simulink model "PX4_Run_Mode_R2017b"  (R2017b)
settings: Solver=FixedStepDiscrete  StartTime=0.0  StopTime=10.0  RelTol=1e-3  EnableMultiTasking=on
InitFcn:
  | run('InitFcn_R2017b_no_csc.m');
values from neighbouring files (symbols this model uses):
  A = Pixhawk_CSC.Parameter( {single([diag([1 1 1]) Ts*diag([1 1 1]); diag([0 0 0]) diag([1 1 1])]),'A'} )    [InitFcn.m]    (also in InitFcn_R2016b.m; InitFcn_R2017b_no_csc.m = single([diag([1 1 1]) Ts*diag([1 1 1]); diag([0 0 0]) diag([)
  app = Pixhawk_CSC.Parameter({single( [0.05; 0.05; 0.05]),'app'} )    [InitFcn.m]    (also in InitFcn_R2016b.m; InitFcn_R2017b_no_csc.m = single( [0.05; 0.05; 0.05]))
  B = Pixhawk_CSC.Parameter( {single([Ts^2/2*diag([1 1 1]); Ts*diag([1 1 1])]),'B'} )    [InitFcn.m]    (also in InitFcn_R2016b.m; InitFcn_R2017b_no_csc.m = single([Ts^2/2*diag([1 1 1]); Ts*diag([1 1 1])]))
  Beta = Pixhawk_CSC.Parameter({single( 0.02),'Beta'} )    [InitFcn.m]    (also in InitFcn_R2016b.m; InitFcn_R2017b_no_csc.m = single( 0.02))
  C = Pixhawk_CSC.Parameter( {single([diag([1 1 1]) 0*diag([1 1 1]); zeros(1,2) 1 zeros(1,3)]),'C'} )    [InitFcn.m]    (also in InitFcn_R2016b.m; InitFcn_R2017b_no_csc.m = single([diag([1 1 1]) 0*diag([1 1 1]); zeros(1,2) 1 zeros(1,)
  C1 = Pixhawk_CSC.Parameter({single( 1.08680),'C1'} )    [InitFcn.m]    (also in InitFcn_R2016b.m; InitFcn_R2017b_no_csc.m = single( 1.08680))
  C10 = Pixhawk_CSC.Parameter({single( 0.0000),'C10'} )    [InitFcn.m]    (also in InitFcn_R2016b.m; InitFcn_R2017b_no_csc.m = single( 0.0000))
  C11 = Pixhawk_CSC.Parameter({single(-0.2300),'C11'} )    [InitFcn.m]    (also in InitFcn_R2016b.m; InitFcn_R2017b_no_csc.m = single(-0.2300))
  C12 = Pixhawk_CSC.Parameter({single( 0.0000),'C12'} )    [InitFcn.m]    (also in InitFcn_R2016b.m; InitFcn_R2017b_no_csc.m = single( 0.0000))
  C13 = Pixhawk_CSC.Parameter({single( 0.8000),'C13'} )    [InitFcn.m]    (also in InitFcn_R2016b.m; InitFcn_R2017b_no_csc.m = single( 0.8000))
  C14 = Pixhawk_CSC.Parameter({single( 0.8000),'C14'} )    [InitFcn.m]    (also in InitFcn_R2016b.m; InitFcn_R2017b_no_csc.m = single( 0.8000))
  C15 = Pixhawk_CSC.Parameter({single( 1.73200),'C15'} )    [InitFcn.m]    (also in InitFcn_R2016b.m; InitFcn_R2017b_no_csc.m = single( 1.73200))
  C16 = Pixhawk_CSC.Parameter({single( 0.1000),'C16'} )    [InitFcn.m]    (also in InitFcn_R2016b.m; InitFcn_R2017b_no_csc.m = single( 0.1000))
  C17 = Pixhawk_CSC.Parameter({single( 0.1000),'C17'} )    [InitFcn.m]    (also in InitFcn_R2016b.m; InitFcn_R2017b_no_csc.m = single( 0.1000))
  C18 = Pixhawk_CSC.Parameter({single( 0.0500),'C18'} )    [InitFcn.m]    (also in InitFcn_R2016b.m; InitFcn_R2017b_no_csc.m = single( 0.0500))
  C19 = Pixhawk_CSC.Parameter({single( 0.6000),'C19'} )    [InitFcn.m]    (also in InitFcn_R2016b.m; InitFcn_R2017b_no_csc.m = single( 0.6000))
  C2 = Pixhawk_CSC.Parameter({single( 1.10468),'C2'} )    [InitFcn.m]    (also in InitFcn_R2016b.m; InitFcn_R2017b_no_csc.m = single( 1.10468))
  C20 = Pixhawk_CSC.Parameter({single( 0.6000),'C20'} )    [InitFcn.m]    (also in InitFcn_R2016b.m; InitFcn_R2017b_no_csc.m = single( 0.6000))
  C21 = Pixhawk_CSC.Parameter({single( 1.04558),'C21'} )    [InitFcn.m]    (also in InitFcn_R2016b.m; InitFcn_R2017b_no_csc.m = single( 1.04558))
  C22 = Pixhawk_CSC.Parameter({single( 0.0000),'C22'} )    [InitFcn.m]    (also in InitFcn_R2016b.m; InitFcn_R2017b_no_csc.m = single( 0.0000))
  C23 = Pixhawk_CSC.Parameter({single( 0.0000),'C23'} )    [InitFcn.m]    (also in InitFcn_R2016b.m; InitFcn_R2017b_no_csc.m = single( 0.0000))
  C24 = Pixhawk_CSC.Parameter({single(-11.0000),'C24'} )    [InitFcn.m]    (also in InitFcn_R2016b.m; InitFcn_R2017b_no_csc.m = single(-11.0000))
  C3 = Pixhawk_CSC.Parameter({single( 1.1980),'C3'} )    [InitFcn.m]    (also in InitFcn_R2016b.m; InitFcn_R2017b_no_csc.m = single( 1.1980))
  C4 = Pixhawk_CSC.Parameter({single( 0.0500),'C4'} )    [InitFcn.m]    (also in InitFcn_R2016b.m; InitFcn_R2017b_no_csc.m = single( 0.0500))
  C5 = Pixhawk_CSC.Parameter({single( 0.0500),'C5'} )    [InitFcn.m]    (also in InitFcn_R2016b.m; InitFcn_R2017b_no_csc.m = single( 0.0500))
  C6 = Pixhawk_CSC.Parameter({single( 0.0500),'C6'} )    [InitFcn.m]    (also in InitFcn_R2016b.m; InitFcn_R2017b_no_csc.m = single( 0.0500))
  C7 = Pixhawk_CSC.Parameter({single( 0.35937),'C7'} )    [InitFcn.m]    (also in InitFcn_R2016b.m; InitFcn_R2017b_no_csc.m = single( 0.35937))
  C8 = Pixhawk_CSC.Parameter({single( 0.36528),'C8'} )    [InitFcn.m]    (also in InitFcn_R2016b.m; InitFcn_R2017b_no_csc.m = single( 0.36528))
  C9 = Pixhawk_CSC.Parameter({single( 0.53311),'C9'} )    [InitFcn.m]    (also in InitFcn_R2016b.m; InitFcn_R2017b_no_csc.m = single( 0.53311))
  C_1 = Pixhawk_CSC.Parameter( {single([diag([1 1 1]) 0*diag([1 1 1])]),'C1'} )    [InitFcn.m]    (also in InitFcn_R2016b.m; InitFcn_R2017b_no_csc.m = single([diag([1 1 1]) 0*diag([1 1 1])]))
  CAL_ACC0_XOFFSET = Pixhawk_CSC.Parameter( {single( 0.122052  ),'CAL_ACC0_XOFFSET'} )    [InitFcn.m]    (also in InitFcn_R2016b.m; InitFcn_R2017b_no_csc.m = single( 0.122052  ))
  CAL_ACC0_XXSCALE = Pixhawk_CSC.Parameter( {single(  1.01218    ),'CAL_ACC0_XXSCALE'} )    [InitFcn.m]    (also in InitFcn_R2016b.m; InitFcn_R2017b_no_csc.m = single(  1.01218    ))
  CAL_ACC0_XYSCALE = Pixhawk_CSC.Parameter( {single( -0.00443301 ),'CAL_ACC0_XYSCALE'} )    [InitFcn.m]    (also in InitFcn_R2016b.m; InitFcn_R2017b_no_csc.m = single( -0.00443301 ))
  CAL_ACC0_XZSCALE = Pixhawk_CSC.Parameter( {single( -0.00505793 ),'CAL_ACC0_XZSCALE'} )    [InitFcn.m]    (also in InitFcn_R2016b.m; InitFcn_R2017b_no_csc.m = single( -0.00505793 ))
  CAL_ACC0_YOFFSET = Pixhawk_CSC.Parameter( {single( 0.00281205),'CAL_ACC0_YOFFSET'} )    [InitFcn.m]    (also in InitFcn_R2016b.m; InitFcn_R2017b_no_csc.m = single( 0.00281205))
  CAL_ACC0_YXSCALE = Pixhawk_CSC.Parameter( {single( -0.00443301 ),'CAL_ACC0_YXSCALE'} )    [InitFcn.m]    (also in InitFcn_R2016b.m; InitFcn_R2017b_no_csc.m = single( -0.00443301 ))
  CAL_ACC0_YYSCALE = Pixhawk_CSC.Parameter( {single(  1.00234    ),'CAL_ACC0_YYSCALE'} )    [InitFcn.m]    (also in InitFcn_R2016b.m; InitFcn_R2017b_no_csc.m = single(  1.00234    ))
  CAL_ACC0_YZSCALE = Pixhawk_CSC.Parameter( {single(  0.0160883  ),'CAL_ACC0_YZSCALE'} )    [InitFcn.m]    (also in InitFcn_R2016b.m; InitFcn_R2017b_no_csc.m = single(  0.0160883  ))
  CAL_ACC0_ZOFFSET = Pixhawk_CSC.Parameter( {single(-0.0298121 ),'CAL_ACC0_ZOFFSET'} )    [InitFcn.m]    (also in InitFcn_R2016b.m; InitFcn_R2017b_no_csc.m = single(-0.0298121 ))
  CAL_ACC0_ZXSCALE = Pixhawk_CSC.Parameter( {single( -0.00505793 ),'CAL_ACC0_ZXSCALE'} )    [InitFcn.m]    (also in InitFcn_R2016b.m; InitFcn_R2017b_no_csc.m = single( -0.00505793 ))
  CAL_ACC0_ZYSCALE = Pixhawk_CSC.Parameter( {single(  0.0160883  ),'CAL_ACC0_ZYSCALE'} )    [InitFcn.m]    (also in InitFcn_R2016b.m; InitFcn_R2017b_no_csc.m = single(  0.0160883  ))
  CAL_ACC0_ZZSCALE = Pixhawk_CSC.Parameter( {single(  0.983604   ),'CAL_ACC0_ZZSCALE'} )    [InitFcn.m]    (also in InitFcn_R2016b.m; InitFcn_R2017b_no_csc.m = single(  0.983604   ))
  CAL_BAR_OFFSET = Pixhawk_CSC.Parameter( {single( -20.8468),'CAL_BAR_OFFSET'} )    [InitFcn.m]    (also in InitFcn_R2016b.m; InitFcn_R2017b_no_csc.m = single( -20.8468))
  CAL_BAR_SCALE = Pixhawk_CSC.Parameter( {single(   1.0632),'CAL_BAR_SCALE'} )    [InitFcn.m]    (also in InitFcn_R2016b.m; InitFcn_R2017b_no_csc.m = single(   1.0632))
  CAL_BAT0_XOFFSET = Pixhawk_CSC.Parameter( {single( 0.0000),'CAL_BAT0_XOFFSET'} )    [InitFcn.m]    (also in InitFcn_R2016b.m; InitFcn_R2017b_no_csc.m = single( 0.0000))
  CAL_BAT0_XXSCALE = Pixhawk_CSC.Parameter( {single(  1.0000),'CAL_BAT0_XXSCALE'} )    [InitFcn.m]    (also in InitFcn_R2016b.m; InitFcn_R2017b_no_csc.m = single(  1.0000))
  CAL_BAT0_XYSCALE = Pixhawk_CSC.Parameter( {single(  0.0000),'CAL_BAT0_XYSCALE'} )    [InitFcn.m]    (also in InitFcn_R2016b.m; InitFcn_R2017b_no_csc.m = single(  0.0000))
  CAL_BAT0_XZSCALE = Pixhawk_CSC.Parameter( {single(  0.0000),'CAL_BAT0_XZSCALE'} )    [InitFcn.m]    (also in InitFcn_R2016b.m; InitFcn_R2017b_no_csc.m = single(  0.0000))
  CAL_BAT0_YOFFSET = Pixhawk_CSC.Parameter( {single( 0.0000),'CAL_BAT0_YOFFSET'} )    [InitFcn.m]    (also in InitFcn_R2016b.m; InitFcn_R2017b_no_csc.m = single( 0.0000))
  CAL_BAT0_YXSCALE = Pixhawk_CSC.Parameter( {single(  0.0000),'CAL_BAT0_YXSCALE'} )    [InitFcn.m]    (also in InitFcn_R2016b.m; InitFcn_R2017b_no_csc.m = single(  0.0000))
  CAL_BAT0_YYSCALE = Pixhawk_CSC.Parameter( {single(  1.0000),'CAL_BAT0_YYSCALE'} )    [InitFcn.m]    (also in InitFcn_R2016b.m; InitFcn_R2017b_no_csc.m = single(  1.0000))
  CAL_BAT0_YZSCALE = Pixhawk_CSC.Parameter( {single(  0.0000),'CAL_BAT0_YZSCALE'} )    [InitFcn.m]    (also in InitFcn_R2016b.m; InitFcn_R2017b_no_csc.m = single(  0.0000))
  CAL_BAT0_ZOFFSET = Pixhawk_CSC.Parameter( {single( 0.0000),'CAL_BAT0_ZOFFSET'} )    [InitFcn.m]    (also in InitFcn_R2016b.m; InitFcn_R2017b_no_csc.m = single( 0.0000))
  CAL_BAT0_ZXSCALE = Pixhawk_CSC.Parameter( {single(  0.0000),'CAL_BAT0_ZXSCALE'} )    [InitFcn.m]    (also in InitFcn_R2016b.m; InitFcn_R2017b_no_csc.m = single(  0.0000))
  CAL_BAT0_ZYSCALE = Pixhawk_CSC.Parameter( {single(  0.0000),'CAL_BAT0_ZYSCALE'} )    [InitFcn.m]    (also in InitFcn_R2016b.m; InitFcn_R2017b_no_csc.m = single(  0.0000))
  CAL_BAT0_ZZSCALE = Pixhawk_CSC.Parameter( {single(  1.0000),'CAL_BAT0_ZZSCALE'} )    [InitFcn.m]    (also in InitFcn_R2016b.m; InitFcn_R2017b_no_csc.m = single(  1.0000))
  CAL_GPS0_XOFFSET = Pixhawk_CSC.Parameter( {single( 0.0000),'CAL_GPS0_XOFFSET'} )    [InitFcn.m]    (also in InitFcn_R2016b.m; InitFcn_R2017b_no_csc.m = single( 0.0000))
  CAL_GPS0_XXSCALE = Pixhawk_CSC.Parameter( {single(  0.0100),'CAL_GPS0_XXSCALE'} )    [InitFcn.m]    (also in InitFcn_R2016b.m; InitFcn_R2017b_no_csc.m = single(  0.0100))
  CAL_GPS0_XYSCALE = Pixhawk_CSC.Parameter( {single(  0.0000),'CAL_GPS0_XYSCALE'} )    [InitFcn.m]    (also in InitFcn_R2016b.m; InitFcn_R2017b_no_csc.m = single(  0.0000))
  CAL_GPS0_XZSCALE = Pixhawk_CSC.Parameter( {single(  0.0000),'CAL_GPS0_XZSCALE'} )    [InitFcn.m]    (also in InitFcn_R2016b.m; InitFcn_R2017b_no_csc.m = single(  0.0000))
  CAL_GPS0_YOFFSET = Pixhawk_CSC.Parameter( {single( 0.0000),'CAL_GPS0_YOFFSET'} )    [InitFcn.m]    (also in InitFcn_R2016b.m; InitFcn_R2017b_no_csc.m = single( 0.0000))
  CAL_GPS0_YXSCALE = Pixhawk_CSC.Parameter( {single(  0.0000),'CAL_GPS0_YXSCALE'} )    [InitFcn.m]    (also in InitFcn_R2016b.m; InitFcn_R2017b_no_csc.m = single(  0.0000))
  CAL_GPS0_YYSCALE = Pixhawk_CSC.Parameter( {single(  0.0100),'CAL_GPS0_YYSCALE'} )    [InitFcn.m]    (also in InitFcn_R2016b.m; InitFcn_R2017b_no_csc.m = single(  0.0100))
  CAL_GPS0_YZSCALE = Pixhawk_CSC.Parameter( {single(  0.0000),'CAL_GPS0_YZSCALE'} )    [InitFcn.m]    (also in InitFcn_R2016b.m; InitFcn_R2017b_no_csc.m = single(  0.0000))
  CAL_GPS0_ZOFFSET = Pixhawk_CSC.Parameter( {single( 0.0000),'CAL_GPS0_ZOFFSET'} )    [InitFcn.m]    (also in InitFcn_R2016b.m; InitFcn_R2017b_no_csc.m = single( 0.0000))
  CAL_GPS0_ZXSCALE = Pixhawk_CSC.Parameter( {single(  0.0000),'CAL_GPS0_ZXSCALE'} )    [InitFcn.m]    (also in InitFcn_R2016b.m; InitFcn_R2017b_no_csc.m = single(  0.0000))
  CAL_GPS0_ZYSCALE = Pixhawk_CSC.Parameter( {single(  0.0000),'CAL_GPS0_ZYSCALE'} )    [InitFcn.m]    (also in InitFcn_R2016b.m; InitFcn_R2017b_no_csc.m = single(  0.0000))
  CAL_GPS0_ZZSCALE = Pixhawk_CSC.Parameter( {single( -0.0010),'CAL_GPS0_ZZSCALE'} )    [InitFcn.m]    (also in InitFcn_R2016b.m; InitFcn_R2017b_no_csc.m = single( -0.0010))
  CAL_GYRO0_XXSCALE = Pixhawk_CSC.Parameter( {single(0.992736),'CAL_GYRO0_XXSCALE'} )    [InitFcn.m]    (also in InitFcn_R2016b.m; InitFcn_R2017b_no_csc.m = single(0.992736))
  CAL_GYRO0_XYSCALE = Pixhawk_CSC.Parameter( {single(0.0000),'CAL_GYRO0_XYSCALE'} )    [InitFcn.m]    (also in InitFcn_R2016b.m; InitFcn_R2017b_no_csc.m = single(0.0000))
  CAL_GYRO0_XZSCALE = Pixhawk_CSC.Parameter( {single(0.0000),'CAL_GYRO0_XZSCALE'} )    [InitFcn.m]    (also in InitFcn_R2016b.m; InitFcn_R2017b_no_csc.m = single(0.0000))
  CAL_GYRO0_YXSCALE = Pixhawk_CSC.Parameter( {single(0.0000),'CAL_GYRO0_YXSCALE'} )    [InitFcn.m]    (also in InitFcn_R2016b.m; InitFcn_R2017b_no_csc.m = single(0.0000))
  CAL_GYRO0_YYSCALE = Pixhawk_CSC.Parameter( {single(1.01609),'CAL_GYRO0_YYSCALE'} )    [InitFcn.m]    (also in InitFcn_R2016b.m; InitFcn_R2017b_no_csc.m = single(1.01609))
  CAL_GYRO0_YZSCALE = Pixhawk_CSC.Parameter( {single(0.0000),'CAL_GYRO0_YZSCALE'} )    [InitFcn.m]    (also in InitFcn_R2016b.m; InitFcn_R2017b_no_csc.m = single(0.0000))
  CAL_GYRO0_ZXSCALE = Pixhawk_CSC.Parameter( {single(0.0000),'CAL_GYRO0_ZXSCALE'} )    [InitFcn.m]    (also in InitFcn_R2016b.m; InitFcn_R2017b_no_csc.m = single(0.0000))
  CAL_GYRO0_ZYSCALE = Pixhawk_CSC.Parameter( {single(0.0000),'CAL_GYRO0_ZYSCALE'} )    [InitFcn.m]    (also in InitFcn_R2016b.m; InitFcn_R2017b_no_csc.m = single(0.0000))
  CAL_GYRO0_ZZSCALE = Pixhawk_CSC.Parameter( {single(1.03003),'CAL_GYRO0_ZZSCALE'} )    [InitFcn.m]    (also in InitFcn_R2016b.m; InitFcn_R2017b_no_csc.m = single(1.03003))
  CAL_MAG0_XCURCOR = Pixhawk_CSC.Parameter( {single( 0.0017     ),'CAL_MAG0_XCURCOR'} )    [InitFcn.m]    (also in InitFcn_R2016b.m; InitFcn_R2017b_no_csc.m = single( 0.0017     ))
  CAL_MAG0_XOFFSET = Pixhawk_CSC.Parameter( {single( 0.0446372  ),'CAL_MAG0_XOFFSET'} )    [InitFcn.m]    (also in InitFcn_R2016b.m; InitFcn_R2017b_no_csc.m = single( 0.0446372  ))
  CAL_MAG0_XXSCALE = Pixhawk_CSC.Parameter( {single(  1.01563   ),'CAL_MAG0_XXSCALE'} )    [InitFcn.m]    (also in InitFcn_R2016b.m; InitFcn_R2017b_no_csc.m = single(  1.01563   ))
  CAL_MAG0_XYSCALE = Pixhawk_CSC.Parameter( {single( -0.0612061 ),'CAL_MAG0_XYSCALE'} )    [InitFcn.m]    (also in InitFcn_R2016b.m; InitFcn_R2017b_no_csc.m = single( -0.0612061 ))
  CAL_MAG0_XZSCALE = Pixhawk_CSC.Parameter( {single( -0.011532  ),'CAL_MAG0_XZSCALE'} )    [InitFcn.m]    (also in InitFcn_R2016b.m; InitFcn_R2017b_no_csc.m = single( -0.011532  ))
  CAL_MAG0_YCURCOR = Pixhawk_CSC.Parameter( {single(-0.0075     ),'CAL_MAG0_YCURCOR'} )    [InitFcn.m]    (also in InitFcn_R2016b.m; InitFcn_R2017b_no_csc.m = single(-0.0075     ))
  CAL_MAG0_YOFFSET = Pixhawk_CSC.Parameter( {single( 0.0700776  ),'CAL_MAG0_YOFFSET'} )    [InitFcn.m]    (also in InitFcn_R2016b.m; InitFcn_R2017b_no_csc.m = single( 0.0700776  ))
  CAL_MAG0_YXSCALE = Pixhawk_CSC.Parameter( {single( -0.0612061 ),'CAL_MAG0_YXSCALE'} )    [InitFcn.m]    (also in InitFcn_R2016b.m; InitFcn_R2017b_no_csc.m = single( -0.0612061 ))
  CAL_MAG0_YYSCALE = Pixhawk_CSC.Parameter( {single(  1.00593   ),'CAL_MAG0_YYSCALE'} )    [InitFcn.m]    (also in InitFcn_R2016b.m; InitFcn_R2017b_no_csc.m = single(  1.00593   ))
  CAL_MAG0_YZSCALE = Pixhawk_CSC.Parameter( {single(  0.0144582 ),'CAL_MAG0_YZSCALE'} )    [InitFcn.m]    (also in InitFcn_R2016b.m; InitFcn_R2017b_no_csc.m = single(  0.0144582 ))
  CAL_MAG0_ZCURCOR = Pixhawk_CSC.Parameter( {single(-0.0080     ),'CAL_MAG0_ZCURCOR'} )    [InitFcn.m]    (also in InitFcn_R2016b.m; InitFcn_R2017b_no_csc.m = single(-0.0080     ))
  CAL_MAG0_ZOFFSET = Pixhawk_CSC.Parameter( {single( 0.00201742 ),'CAL_MAG0_ZOFFSET'} )    [InitFcn.m]    (also in InitFcn_R2016b.m; InitFcn_R2017b_no_csc.m = single( 0.00201742 ))
  CAL_MAG0_ZXSCALE = Pixhawk_CSC.Parameter( {single( -0.011532  ),'CAL_MAG0_ZXSCALE'} )    [InitFcn.m]    (also in InitFcn_R2016b.m; InitFcn_R2017b_no_csc.m = single( -0.011532  ))
  CAL_MAG0_ZYSCALE = Pixhawk_CSC.Parameter( {single(  0.0144582 ),'CAL_MAG0_ZYSCALE'} )    [InitFcn.m]    (also in InitFcn_R2016b.m; InitFcn_R2017b_no_csc.m = single(  0.0144582 ))
  CAL_MAG0_ZZSCALE = Pixhawk_CSC.Parameter( {single(  0.986813  ),'CAL_MAG0_ZZSCALE'} )    [InitFcn.m]    (also in InitFcn_R2016b.m; InitFcn_R2017b_no_csc.m = single(  0.986813  ))
  CAL_SONAR_OFFSET = Pixhawk_CSC.Parameter( {single( -6.8730),'CAL_SONAR_OFFSET'} )    [InitFcn.m]    (also in InitFcn_R2016b.m; InitFcn_R2017b_no_csc.m = single( -6.8730))
  CAL_SONAR_SCALE = Pixhawk_CSC.Parameter( {single(-438.1875),'CAL_SONAR_SCALE'} )    [InitFcn.m]    (also in InitFcn_R2016b.m; InitFcn_R2017b_no_csc.m = single(-438.1875))
  COM_RATE = double(10)    [InitFcn.m]    (also in InitFcn_R2016b.m; InitFcn_R2017b_no_csc.m)
  D = Pixhawk_CSC.Parameter( {single(zeros(size(C.Value,1), size(B.Value,2))),'D'} )    [InitFcn.m]    (also in InitFcn_R2016b.m; InitFcn_R2017b_no_csc.m = single(zeros(size(C,1), size(B,2))))
  Dip0 = Pixhawk_CSC.Parameter({single( 1.2),'Dip0'} )    [InitFcn.m]    (also in InitFcn_R2016b.m; InitFcn_R2017b_no_csc.m = single( 1.2))
  I = Pixhawk_CSC.Parameter( {single(eye(size(Q.Value))),'I'} )    [InitFcn.m]    (also in InitFcn_R2016b.m; InitFcn_R2017b_no_csc.m = single(eye(size(Q))))
  Jxx = Pixhawk_CSC.Parameter( {single(J(1,1)),'Jxx'} )    [InitFcn.m]    (also in InitFcn_R2016b.m; InitFcn_R2017b_no_csc.m = single(J(1,1)))
  Jyy = Pixhawk_CSC.Parameter( {single(J(2,2)),'Jyy'} )    [InitFcn.m]    (also in InitFcn_R2016b.m; InitFcn_R2017b_no_csc.m = single(J(2,2)))
  Jzz = Pixhawk_CSC.Parameter( {single(J(3,3)),'Jzz'} )    [InitFcn.m]    (also in InitFcn_R2016b.m; InitFcn_R2017b_no_csc.m = single(J(3,3)))
  Kapp = Pixhawk_CSC.Parameter({single( 1.2),'Kapp'} )    [InitFcn.m]    (also in InitFcn_R2016b.m; InitFcn_R2017b_no_csc.m = single( 1.2))
  Kx = Pixhawk_CSC.Parameter({single( Kx),'Kx'} )    [InitFcn.m]    (also in InitFcn_R2016b.m = Pixhawk_CSC.Parameter({single( [0.60 0.9]),'Kx'} ); InitFcn_R2017b_no_csc.m = single( [0.60 0.9]))
  Ky = Pixhawk_CSC.Parameter({single( Ky),'Ky'} )    [InitFcn.m]    (also in InitFcn_R2016b.m = Pixhawk_CSC.Parameter({single( [0.4 0.9]),'Ky'} ); InitFcn_R2017b_no_csc.m = single( [0.4 0.9]))
  LPF_REF_DEN = Pixhawk_CSC.Parameter( {single([1.0000 -0.8187]),'LPF_REF_DEN'} )    [InitFcn.m]    (also in InitFcn_R2016b.m; InitFcn_R2017b_no_csc.m = single([1.0000 -0.8187]))
  LPF_REF_NUM = Pixhawk_CSC.Parameter( {single([0.0000  0.1813]),'LPF_REF_NUM'} )    [InitFcn.m]    (also in InitFcn_R2016b.m; InitFcn_R2017b_no_csc.m = single([0.0000  0.1813]))
  m0 = Pixhawk_CSC.Parameter({single( 0.452857),'m0'} )    [InitFcn.m]    (also in InitFcn_R2016b.m; InitFcn_R2017b_no_csc.m = single( 0.452857))
  mn = [0.01; 0.01; 0.01; 0.01]    [InitFcn.m]    (also in InitFcn_R2016b.m; InitFcn_R2017b_no_csc.m)
  MOV_AVG_WINDOW = Pixhawk_CSC.Parameter( {single(100),'MOV_AVG_WINDOW'} )    [InitFcn.m]    (also in InitFcn_R2016b.m; InitFcn_R2017b_no_csc.m = single(100))
  Ox0 = Pixhawk_CSC.Parameter({single(O_x0),'Ox0'} )    [InitFcn.m]    (also in InitFcn_R2016b.m; InitFcn_R2017b_no_csc.m = single(O_x0))
  Oxa = Pixhawk_CSC.Parameter({single(O_x.a),'Oxa'} )    [InitFcn.m]    (also in InitFcn_R2016b.m; InitFcn_R2017b_no_csc.m = single(O_x.a))
  Oxb = Pixhawk_CSC.Parameter({single(O_x.b),'Oxb'} )    [InitFcn.m]    (also in InitFcn_R2016b.m; InitFcn_R2017b_no_csc.m = single(O_x.b))
  Oxc = Pixhawk_CSC.Parameter({single(O_x.c),'Oxc'} )    [InitFcn.m]    (also in InitFcn_R2016b.m; InitFcn_R2017b_no_csc.m = single(O_x.c))
  Oxd = Pixhawk_CSC.Parameter({single(O_x.d),'Oxd'} )    [InitFcn.m]    (also in InitFcn_R2016b.m; InitFcn_R2017b_no_csc.m = single(O_x.d))
  Oy0 = Pixhawk_CSC.Parameter({single(O_y0),'Oy0'} )    [InitFcn.m]    (also in InitFcn_R2016b.m; InitFcn_R2017b_no_csc.m = single(O_y0))
  Oya = Pixhawk_CSC.Parameter({single(O_y.a),'Oya'} )    [InitFcn.m]    (also in InitFcn_R2016b.m; InitFcn_R2017b_no_csc.m = single(O_y.a))
  Oyb = Pixhawk_CSC.Parameter({single(O_y.b),'Oyb'} )    [InitFcn.m]    (also in InitFcn_R2016b.m; InitFcn_R2017b_no_csc.m = single(O_y.b))
  Oyc = Pixhawk_CSC.Parameter({single(O_y.c),'Oyc'} )    [InitFcn.m]    (also in InitFcn_R2016b.m; InitFcn_R2017b_no_csc.m = single(O_y.c))
  Oyd = Pixhawk_CSC.Parameter({single(O_y.d),'Oyd'} )    [InitFcn.m]    (also in InitFcn_R2016b.m; InitFcn_R2017b_no_csc.m = single(O_y.d))
  Oz0 = Pixhawk_CSC.Parameter({single(O_z0),'Oz0'} )    [InitFcn.m]    (also in InitFcn_R2016b.m; InitFcn_R2017b_no_csc.m = single(O_z0))
  ... (+53 more)
undefined symbols (not defined in the file or in its folder): AccX, AccY, AccZ, Altitude, ax, ay, az, Current, FILTER_N, GPS_TS, GyroX, GyroY, GyroZ, Latitude, Longitude, M1_PWM, M2_PWM, M3_PWM, M4_PWM, MagX, MagY, MagZ, mAH, MOTOR, phi, Position_TS, psi, PX4_TUNE_ENUM, RGBLED_COLOR_ENUM, RGBLED_MODE_ENUM, S_AccX, S_AccY, S_AccZ, S_Altitude, S_Baro, S_Current, S_GyroX, S_GyroY, S_GyroZ, S_Latitude, S_Longitude, S_MagX, S_MagY, S_MagZ, S_mAH, S_N_Sat, S_Voltage, T_PITCH, T_ROLL, T_THROTTLE, theta, v, Voltage, w, wx, wxd, wy, wyd, wz ... (+4)
libraries: simulink x31, pixhawk_slib_sensors_actuators x7, pixhawk_slib_ADC_serial x5, pixhawk_slib_misc_utils x3, etargetslib x2
(part 1 of 7)
Description:
  | PX4 PSP Demo Model - LED
  | 
  | This model shows how to use the LED Output Block.
  | Use this model to prove out the workflow from Code Gen to Hardware.
settings Model: Creator=skuznick  LastModifiedBy=tom
settings SolverCC: PositivePriorityOrder=on
settings DataIOCC: LimitDataPoints=on  SaveFormat=Array
settings OptimizationCC: DefaultParameterBehavior=Inlined  LifeSpan=1  MaxStackSize=64
settings DebuggingCC: SolverPrmCheckMsg=warning  AllowSymbolicDim=off  SFUnexpectedBacktrackingDiag=warning  SFNoUnconditionalDefaultTransitionDiag=warning  SFExecutionAtInitializationDiag=none
settings HardwareCC: ProdBitPerPointer=32  ProdBitPerSizeT=32  ProdBitPerPtrDiffT=32  ProdLargestAtomicInteger=Long  ProdLargestAtomicFloat=Double  ProdWordSize=32  ProdHWDeviceType=ARM Compatible->ARM Cortex
settings ModelReferenceCC: PropagateSignalLabelsOutOfModel=off
settings SFSimCC: MATLABDynamicMemAlloc=off
settings RTWCC: SystemTargetFile=ert.tlc  HardwareBoard=Pixhawk PX4  TemplateMakefile=ert_default_tmf  GenerateReport=on  Toolchain=Pixhawk Toolchain  IncludeHyperlinkInReport=on  LaunchReport=on  GenerateTraceReport=on  GenerateCodeMetricsReport=on
settings CodeAppCC: IgnoreCustomStorageClasses=off  StateflowObjectComments=on
settings ERTTargetCC: MultiwordLength=2048  ERTCustomFileTemplate=px4_codertarget_file_process.tlc  ConvertIfToSwitch=off  SuppressUnreachableDefaultCases=off
settings ConfigComp: CovMetricSettings=dw  CovHtmlReporting=on  CovSaveCumulativeToWorkspaceVar=on  CovSaveSingleToWorkspaceVar=on  CovExternalEMLEnable=off  CovSFcnEnable=off

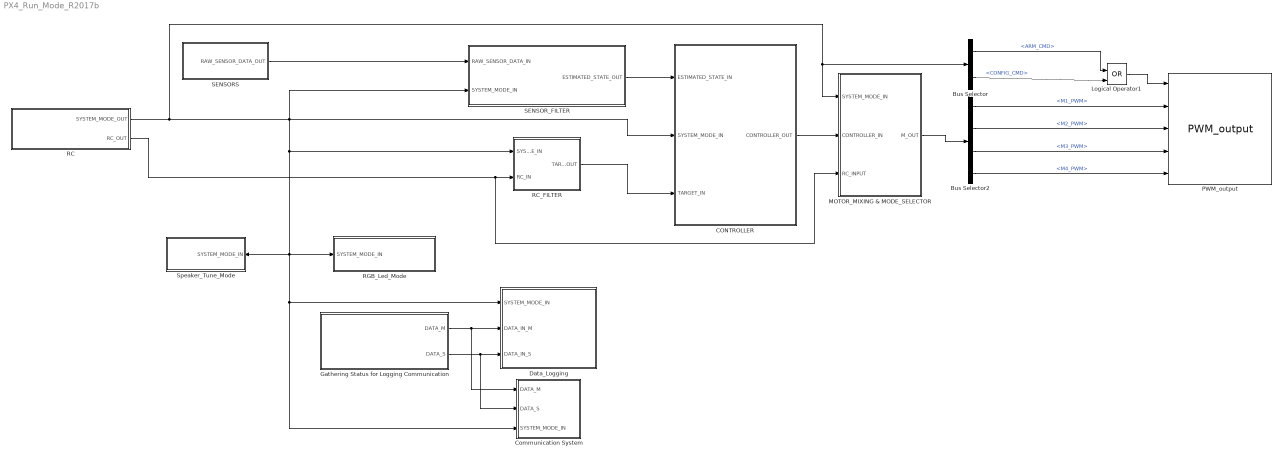
== system PX4_Run_Mode_R2017b ==
  Bus Selector : BusSelector  OutputSignals=ARM_CMD,CONFIG_CMD
  Bus Selector2 : BusSelector  OutputSignals=M1_PWM,M2_PWM,M3_PWM,M4_PWM
  CONTROLLER : Subsystem
  Communication System : Subsystem
  Data_Logging : Subsystem
  Gathering Status for Logging Communication : Subsystem
  Logical Operator1 : Logic  Operator=OR  IconShape=distinctive  AllPortsSameDT=off  OutDataTypeStr=boolean
  MOTOR_MIXING & MODE_SELECTOR : Subsystem
  PWM_output : pixhawk_slib_sensors_actuators/PWM_output  pub_outputs=on  pwm_rate=400Hz  show_pwm1=on  show_pwm5=off  show_pwm2=on  show_pwm6=off  show_pwm3=on  show_pwm7=off  show_pwm4=on  show_pwm8=off
      settings: SourceProductName=Pixhawk Target Blocks
  RC : Subsystem
  RC_FILTER : Subsystem
  RGB_Led_Mode : Subsystem
  SENSORS : Subsystem
  SENSOR_FILTER : Subsystem
  Speaker_Tune_Mode : Subsystem
  wires:
  Bus Selector2/1 -> PWM_output/2  "<M1_PWM>"
  SENSORS/1(RAW_SENSOR_DATA_OUT) -> SENSOR_FILTER/1(RAW_SENSOR_DATA_IN)
  Bus Selector2/2 -> PWM_output/3  "<M2_PWM>"
  CONTROLLER/1(CONTROLLER_OUT) -> MOTOR_MIXING & MODE_SELECTOR/2(CONTROLLER_IN)
  Bus Selector2/4 -> PWM_output/5  "<M4_PWM>"
  Bus Selector/2 -> Logical Operator1/2  "<CONFIG_CMD>"
  Bus Selector/1 -> Logical Operator1/1  "<ARM_CMD>"
  Gathering Status for Logging Communication/2(DATA_S) -> Data_Logging/3(DATA_IN_S), Communication System/2(DATA_S)
  Logical Operator1/1 -> PWM_output/1
  RC_FILTER/1(TARGET_OUT) -> CONTROLLER/3(TARGET_IN)
  Gathering Status for Logging Communication/1(DATA_M) -> Data_Logging/2(DATA_IN_M), Communication System/1(DATA_M)
  RC/2(RC_OUT) -> MOTOR_MIXING & MODE_SELECTOR/3(RC_INPUT), RC_FILTER/2(RC_IN)
  Bus Selector2/3 -> PWM_output/4  "<M3_PWM>"
  RC/1(SYSTEM_MODE_OUT) -> RGB_Led_Mode/1(SYSTEM_MODE_IN), Communication System/3(SYSTEM_MODE_IN), Data_Logging/1(SYSTEM_MODE_IN), Speaker_Tune_Mode/1(SYSTEM_MODE_IN), RC_FILTER/1(SYSTEM_MODE_IN), CONTROLLER/2(SYSTEM_MODE_IN), SENSOR_FILTER/2(SYSTEM_MODE_IN), Bus Selector/1, MOTOR_MIXING & MODE_SELECTOR/1(SYSTEM_MODE_IN)
  MOTOR_MIXING & MODE_SELECTOR/1(M_OUT) -> Bus Selector2/1
  SENSOR_FILTER/1(ESTIMATED_STATE_OUT) -> CONTROLLER/1(ESTIMATED_STATE_IN)

== system PX4_Run_Mode_R2017b/CONTROLLER ==
  ESTIMATED_STATE_IN : Inport
  SYSTEM_MODE_IN : Inport  Port=2
  TARGET_IN : Inport  Port=3
  Bus Creator1 : BusCreator  Inputs=4
  Bus Selector : BusSelector  OutputSignals=T_THROTTLE
  Data Type Conversion{12..15} (4 alike) : DataTypeConversion  OutDataTypeStr=single
  Inner Control Loop : Subsystem
  Outer Control Loop : Subsystem
  Product{,1..3} (4 alike) : Product
  Ramp : Subsystem
  CONTROLLER_OUT : Outport
  tag scope: CONTROLLER=global, ERROR=global
  wires:
  TARGET_IN/1 -> Outer Control Loop/2(TARGET_IN)
  Product1/1 -> Data Type Conversion13/1
  Product2/1 -> Data Type Conversion12/1
  SYSTEM_MODE_IN/1 -> Outer Control Loop/3(SYSTEM_MODE_IN), Inner Control Loop/4("SYSTEM_MODE_IN "), Ramp/1(SYSTEM_MODE_IN)
  Data Type Conversion12/1 -> Bus Creator1/3  "CON_YAW"
  Data Type Conversion13/1 -> Bus Creator1/2  "CON_PITCH"
  Data Type Conversion14/1 -> Bus Creator1/1  "CON_ROLL"
  Data Type Conversion15/1 -> Bus Creator1/4  "CON_THROTTLE"
  Product/1 -> Data Type Conversion14/1
  Bus Creator1/1 -> CONTROLLER_OUT/1, [CONTROLLER]
  ESTIMATED_STATE_IN/1 -> Inner Control Loop/1(ESTIMATED_STATE_IN), Outer Control Loop/1(ESTIMATED_STATE_IN)
  Inner Control Loop/2(U Roll) -> Product/1
  Inner Control Loop/3(U Pitch) -> Product1/1
  Inner Control Loop/4(U Yaw) -> Product2/1
  Ramp/1(RAMP) -> Product/2, Product1/2, Product2/2, Product3/2
  Outer Control Loop/1(TARGET_OUT) -> Bus Selector/1, Inner Control Loop/2(TARGET_IN)
  Bus Selector/1 -> Product3/1  "<T_THROTTLE>"
  Product3/1 -> Data Type Conversion15/1
  Outer Control Loop/2(ERROR_OUT) -> Inner Control Loop/3(ERROR_IN)
  Inner Control Loop/1(ERROR_OUT) -> [ERROR]

== system PX4_Run_Mode_R2017b/Communication System ==
  DATA_M : Inport
  DATA_S : Inport  Port=2
  SYSTEM_MODE_IN : Inport  Port=3
  Bus Selector : BusSelector  OutputSignals=ESTIMATED_STATE.x,ESTIMATED_STATE.y,ESTIMATED_STATE.z,ESTIMATED_STATE.phi,ESTIMATED_STATE.theta,ESTIMATED_STATE.psi,TARGET.T_THROTTLE,TARGET.T_ROLL,TARGET.T_PITCH,TARGET.T_YAW  OutputAsBus=on
  Bus Selector1 : BusSelector  OutputSignals=State Bias Parameters.X_BIAS,State Bias Parameters.Y_BIAS,State Bias Parameters.Z_BIAS,State Bias Parameters.PHI_BIAS,State Bias Parameters.THETA_BIAS,State Bias Parameters.PSI_BIAS  OutputAsBus=on
  Bus Selector2 : BusSelector  OutputSignals=ARM_CMD  OutputAsBus=on
  Bus to Vector : BusToVector
  Bus to Vector1 : BusToVector
  Data Type Conversion5 : DataTypeConversion  OutDataTypeStr=single
  Incomming Communication : Subsystem
  Mux : Mux  Inputs=2
  Outgoining Communication : Subsystem
  Rate Transition : RateTransition  OutPortSampleTime=1/double(COM_RATE)
  Rate Transition4 : RateTransition  OutPortSampleTime=1/double(COM_RATE)
  Rate Transition5 : RateTransition  OutPortSampleTime=Ts
  Set Online Control Gains : Subsystem
  Terminator : Terminator
  Terminator1 : Terminator
  wires:
  DATA_M/1 -> Bus Selector/1
  Bus Selector/1 -> Bus to Vector/1
  Bus to Vector/1 -> Rate Transition/1
  Incomming Communication/2(Control Value) -> Mux/1
  Rate Transition/1 -> Mux/2
  DATA_S/1 -> Bus Selector1/1
  Bus Selector1/1 -> Bus to Vector1/1
  Bus to Vector1/1 -> Rate Transition4/1
  Rate Transition4/1 -> Terminator/1
  Incomming Communication/1(COM_IN) -> Data Type Conversion5/1
  Rate Transition5/1 -> Set Online Control Gains/2(New Gains)
  Data Type Conversion5/1 -> Rate Transition5/1
  SYSTEM_MODE_IN/1 -> Bus Selector2/1
  Mux/1 -> Outgoining Communication/1(COM_OUT)
  Bus Selector2/1 -> Set Online Control Gains/1(System Mode)
  Set Online Control Gains/1(Control Gains) -> Terminator1/1

== system PX4_Run_Mode_R2017b/Data_Logging ==
  note: If System is in Armed mode
      | And not in config mode
      | RC_Config enables datalogging
      |
      | Logging varying signals
  SYSTEM_MODE_IN : Inport
  DATA_IN_M : Inport  Port=2
  DATA_IN_S : Inport  Port=3
  Bus Selector : BusSelector  OutputSignals=RECORDING,CONFIG_CMD
  Bus Selector1 : BusSelector  OutputSignals=RECORDING
  Bus Selector2 : BusSelector  OutputSignals=Kalman Filter Parameters,Control Gains Parameters,RC Parameters,State Limit Parameters,PWM Parameters,Motor Mixing Parameters,State Bias Parameters  OutputAsBus=on
  Bus Selector3 : BusSelector  OutputSignals=General Parameters,Magnetometer Parameters,Accelerometer Parameters,Gyroscope Parameters,Barometer Parameters,GPS Parameters,Battery Parameters,Sonar Parameters,Filter Parameters,Madgewick Filter Parameters  OutputAsBus=on
  Bus to Vector : BusToVector
  Bus to Vector1 : BusToVector
  Bus to Vector2 : BusToVector
  Delay : Delay  DelayLength=1  InitialCondition=0
  Logical Operator : Logic  Operator=NAND  IconShape=distinctive  AllPortsSameDT=off  OutDataTypeStr=boolean
  Logical Operator1 : Logic  IconShape=distinctive  AllPortsSameDT=off  OutDataTypeStr=boolean
  Logical Operator2 : Logic  Operator=OR  IconShape=distinctive  AllPortsSameDT=off  OutDataTypeStr=boolean
  Rate Transition : RateTransition  OutPortSampleTime=1/50
  Rate Transition1 : RateTransition  OutPortSampleTime=1/50
  Rate Transition2 : RateTransition  OutPortSampleTime=1/50
  binary_logger : pixhawk_slib_misc_utils/binary_logger  logfile=/fs/microsd/logging/RawSensorData  cacheflag=off  numRecs=1000
      settings: SourceProductName=Pixhawk Target Blocks
  binary_logger1 : pixhawk_slib_misc_utils/binary_logger  logfile=/fs/microsd/logging/SettingsP1  cacheflag=off  numRecs=1000
      settings: SourceProductName=Pixhawk Target Blocks
  binary_logger2 : pixhawk_slib_misc_utils/binary_logger  logfile=/fs/microsd/logging/SettingsP2  cacheflag=off  numRecs=1000
      settings: SourceProductName=Pixhawk Target Blocks
  wires:
  DATA_IN_M/1 -> Bus to Vector/1
  Bus Selector/1 -> Logical Operator2/1  "<RECORDING>"
  SYSTEM_MODE_IN/1 -> Bus Selector1/1, Bus Selector/1
  Bus Selector1/1 -> Rate Transition/1  "<RECORDING>"
  Delay/1 -> Logical Operator/2
  Logical Operator/1 -> Logical Operator1/2
  Logical Operator1/1 -> binary_logger2/1, binary_logger1/1
  DATA_IN_S/1 -> Bus Selector2/1, Bus Selector3/1
  Bus Selector/2 -> Logical Operator2/2  "<CONFIG_CMD>"
  Logical Operator2/1 -> binary_logger/1
  Bus to Vector/1 -> binary_logger/2
  Bus to Vector1/1 -> binary_logger1/2
  Rate Transition/1 -> Delay/1, Logical Operator/1, Logical Operator1/1
  Rate Transition1/1 -> Bus to Vector1/1
  Bus Selector2/1 -> Rate Transition2/1
  Rate Transition2/1 -> Bus to Vector2/1
  Bus to Vector2/1 -> binary_logger2/2
  Bus Selector3/1 -> Rate Transition1/1

== system PX4_Run_Mode_R2017b/Gathering Status for Logging Communication ==
  Bus Creator : BusCreator  Inputs=11
  ConvertM2Single : Subsystem
  ConvertM2Single1 : Subsystem
  ConvertRC2Single : Subsystem
  DATA_M : Outport
  DATA_S : Outport  Port=2
  wires:
  [TARGET] -> Bus Creator/2  "TARGET"
  [CONTROLLER] -> Bus Creator/7  "CONTROLLER"
  Bus Creator/1 -> DATA_M/1
  [RC] -> ConvertRC2Single/1(RC_IN)  "RC"
  [M] -> ConvertM2Single/1(M_IN)  "M"
  ConvertM2Single/1(M_OUT) -> Bus Creator/8
  ConvertRC2Single/1(RC_OUT) -> Bus Creator/1
  [ESTIMATED_STATE] -> Bus Creator/5  "ESTIMATED_STATE"
  [RAW_SENSOR_DATA] -> Bus Creator/3  "RAW_SENSOR_DATA"
  [CLOCKS] -> Bus Creator/10  "CLOCK"
  [ERROR] -> Bus Creator/6  "ERROR"
  [SYSTEM_MODE] -> ConvertM2Single1/1(SYSTEM_MODE_IN)  "SYSTEM_MODE"
  ConvertM2Single1/1(SYSTEM_MODE_OUT) -> Bus Creator/9  "SYSTEM_MODE"
  [FILTERED_SENSOR_DATA] -> Bus Creator/4  "FILTERED_SENSOR_DATA"
  [PARAMETERS] -> DATA_S/1
  [IMP] -> Bus Creator/11  "IMP"

== system PX4_Run_Mode_R2017b/MOTOR_MIXING & MODE_SELECTOR ==
  SYSTEM_MODE_IN : Inport
  CONTROLLER_IN : Inport  Port=2
  RC_INPUT : Inport  Port=3
  " " : MATLAB Function  TreatAsAtomicUnit=on
  Bus Assignment : BusAssignment  AssignedSignals=M1_PWM,M2_PWM,M3_PWM,M4_PWM,MOTOR
  Bus Creator : BusCreator  Inputs=7
  Bus Selector : BusSelector  OutputSignals=Rc_Thrust
  Bus Selector1 : BusSelector  OutputSignals=M1_PWM,M2_PWM,M3_PWM,M4_PWM
  Bus Selector2 : BusSelector  OutputSignals=CONFIG_CMD,CONFIG_M1,CONFIG_M2,CONFIG_M3,CONFIG_M4
  Bus Selector3 : BusSelector  OutputSignals=CON_THROTTLE,CON_ROLL,CON_PITCH,CON_YAW
  Constant : Constant  Value=0  SampleTime=Ts
  Data Type Conversion{4..10} (7 alike) : DataTypeConversion  OutDataTypeStr=uint16
  Motor Configuration : MATLAB Function  TreatAsAtomicUnit=on
  M_OUT : Outport
  tag scope: M=global
  wires:
  RC_INPUT/1 -> Bus Selector/1
  Bus Assignment/1 -> [M], M_OUT/1
  Bus Creator/1 -> Bus Assignment/1, Bus Selector1/1
  Bus Selector1/1 -> Motor Configuration/1(M1_IN)  "<M1_PWM>"
  Bus Selector1/2 -> Motor Configuration/2(M2_IN)  "<M2_PWM>"
  Bus Selector1/3 -> Motor Configuration/3(M3_IN)  "<M3_PWM>"
  Bus Selector1/4 -> Motor Configuration/4(M4_IN)  "<M4_PWM>"
  Motor Configuration/1(M1_OUT) -> Bus Assignment/2
  Motor Configuration/2(M2_OUT) -> Bus Assignment/3
  Motor Configuration/3(M3_OUT) -> Bus Assignment/4
  Motor Configuration/4(M4_OUT) -> Bus Assignment/5
  SYSTEM_MODE_IN/1 -> Bus Selector2/1
  Bus Selector2/1 -> Motor Configuration/6(CONFIG_CMD_IN)  "<CONFIG_CMD>"
  Motor Configuration/5(Motor) -> Bus Assignment/6
  Bus Selector/1 -> Motor Configuration/5(THRUST)  "<Rc_Thrust>"
  Bus Selector2/5 -> Motor Configuration/10(CONFIG_M4)  "<CONFIG_M4>"
  Bus Selector2/4 -> Motor Configuration/9(CONFIG_M3)  "<CONFIG_M3>"
  Bus Selector2/3 -> Motor Configuration/8(CONFIG_M2)  "<CONFIG_M2>"
  Bus Selector2/2 -> Motor Configuration/7(CONFIG_M1)  "<CONFIG_M1>"
  " "/1(M1) -> Data Type Conversion4/1
  " "/2(M2) -> Data Type Conversion5/1
  " "/3(M3) -> Data Type Conversion6/1
  " "/4(M4) -> Data Type Conversion7/1
  Data Type Conversion4/1 -> Bus Creator/1  "M1_PWM"
  Data Type Conversion5/1 -> Bus Creator/2  "M2_PWM"
  Data Type Conversion6/1 -> Bus Creator/3  "M3_PWM"
  Data Type Conversion7/1 -> Bus Creator/4  "M4_PWM"
  " "/5(type1) -> Data Type Conversion8/1
  Data Type Conversion8/1 -> Bus Creator/5  "SOLVER_TYPE1"
  " "/6(type2) -> Data Type Conversion9/1
  Data Type Conversion9/1 -> Bus Creator/6  "SOLVER_TYPE2"
  Data Type Conversion10/1 -> Bus Creator/7  "MOTOR"
  Constant/1 -> Data Type Conversion10/1
  CONTROLLER_IN/1 -> Bus Selector3/1
  Bus Selector3/2 -> " "/2(Roll)  "<CON_ROLL>"
  Bus Selector3/1 -> " "/1(Thrust)  "<CON_THROTTLE>"
  Bus Selector3/3 -> " "/3(Pitch)  "<CON_PITCH>"
  Bus Selector3/4 -> " "/4(Yaw)  "<CON_YAW>"

== system PX4_Run_Mode_R2017b/RC ==
  Arming : Subsystem
  Auto/Man Flight : Subsystem
  Bus Creator : BusCreator  Inputs=10
  Bus Creator1 : BusCreator  Inputs=11
  Motor Configuration : Subsystem
  Recording Data : Subsystem
  input_rc : pixhawk_slib_sensors_actuators/input_rc  sampletime=Ts  channel1=on  channel2=on  channel3=on  channel4=on  channel5=on  channel6=on  channel7=on  channel8=on  channel9=off  channel10=off  channel11=off  channel12=off  channel13=off  channel14=off  channel15=off  channel16=off  channel17=off  channel18=off  ch_count=off  rssi=on  rc_failsafe=on  rc_lost=off  rc_inputsource=off
      settings: SourceProductName=Pixhawk Target Blocks
  SYSTEM_MODE_OUT : Outport
  RC_OUT : Outport  Port=2
  tag scope: RC=global, SYSTEM_MODE=global
  wires:
  input_rc/1 -> Bus Creator/1  "Rc_Roll"
  input_rc/4 -> Bus Creator/4  "Rc_Thrust"
  input_rc/5 -> Bus Creator/5  "Rc_Arm"
  input_rc/10 -> Bus Creator/10  "Rc_Failsafe"
  input_rc/9 -> Bus Creator/9  "Rc_RSSI"
  input_rc/6 -> Bus Creator/6  "Rc_Config_1"
  input_rc/7 -> Bus Creator/7  "Rc_Config_2"
  input_rc/3 -> Bus Creator/3  "Rc_Pitch"
  input_rc/2 -> Bus Creator/2  "Rc_Yaw"
  Bus Creator/1 -> Motor Configuration/1(RC_INPUT), Recording Data/1(RC_INPUT), Auto/Man Flight/1(RC_INPUT), Arming/1(RC_INPUT), [RC], RC_OUT/1
  Bus Creator1/1 -> SYSTEM_MODE_OUT/1, [SYSTEM_MODE]
  Motor Configuration/1(CONFIG_M1) -> Bus Creator1/8  "CONFIG_M1"
  Motor Configuration/2(CONFIG_M2) -> Bus Creator1/9  "CONFIG_M2"
  Motor Configuration/3(CONFIG_M3) -> Bus Creator1/10  "CONFIG_M3"
  Motor Configuration/4(CONFIG_M4) -> Bus Creator1/11  "CONFIG_M4"
  Recording Data/1(RECORDING) -> Bus Creator1/7  "RECORDING"
  Auto/Man Flight/1(MANUAL_FLIGHT) -> Bus Creator1/4  "MAN_FLIGHT"
  Auto/Man Flight/3(AUTO_FLIGHT) -> Bus Creator1/6  "AUTO_FLIGHT"
  Arming/1(ARM_CMD) -> Bus Creator1/1  "ARM_CMD"
  Arming/2(PRE_ARM_CMD) -> Bus Creator1/2  "PRE_ARM_CMD"
  Arming/3(CONFIG_CMD) -> Bus Creator1/3  "CONFIG_CMD"
  Auto/Man Flight/2(SEMI_AUTO_FLIGHT) -> Bus Creator1/5  "SEMI_AUTO_FLIGHT"
  input_rc/8 -> Bus Creator/8  "RC_Optional"

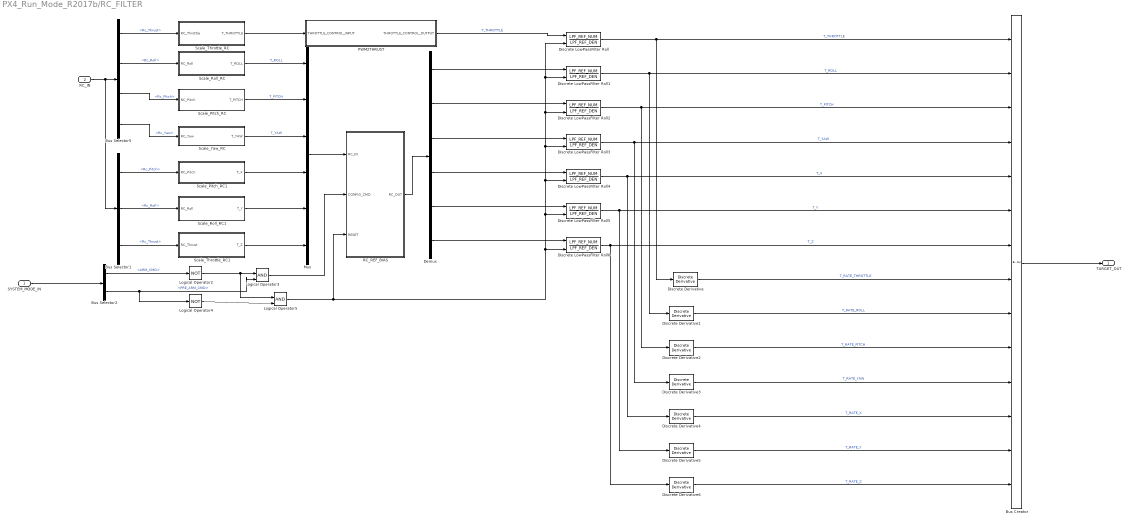
== system PX4_Run_Mode_R2017b/RC_FILTER ==
  SYSTEM_MODE_IN : Inport
  RC_IN : Inport  Port=2
  Bus Creator : BusCreator  Inputs=14
  Bus Selector1 : BusSelector  OutputSignals=Rc_Pitch,Rc_Roll,Rc_Thrust
  Bus Selector2 : BusSelector  OutputSignals=ARM_CMD,PRE_ARM_CMD
  Bus Selector5 : BusSelector  OutputSignals=Rc_Thrust,Rc_Roll,Rc_Pitch,Rc_Yaw
  Demux : Demux  Outputs=6
  Discrete LowPassFilter Roll{,1..6} (7 alike) : DiscreteTransferFcn  Numerator=LPF_REF_NUM  Denominator=LPF_REF_DEN  ExternalReset=Level  SampleTime=Ts
      settings: InputPortMap=u0,r7
  Discrete Derivative{,1..6} (7 alike) : simulink/Discrete/Discrete Derivative  gainval=1.0  ICPrevScaledInput=0.0  OutMin=[]  OutMax=[]  OutDataType=fixdt(1, 16)  OutScaling=2^-10  DoSatur=off
  Logical Operator2 : Logic  Operator=NOT  IconShape=distinctive  AllPortsSameDT=off  OutDataTypeStr=boolean
  Logical Operator3 : Logic  IconShape=distinctive  AllPortsSameDT=off  OutDataTypeStr=boolean
  Logical Operator4 : Logic  Operator=NOT  IconShape=distinctive  AllPortsSameDT=off  OutDataTypeStr=boolean
  Logical Operator5 : Logic  IconShape=distinctive  AllPortsSameDT=off  OutDataTypeStr=boolean
  Mux : Mux  Inputs=6
  PWM2THRUST : MATLAB Function  TreatAsAtomicUnit=on
  RC_REF_BIAS : MATLAB Function  TreatAsAtomicUnit=on
  Scale_Pitch_RC : MATLAB Function  TreatAsAtomicUnit=on
  Scale_Pitch_RC1 : MATLAB Function  TreatAsAtomicUnit=on
  Scale_Roll_RC : MATLAB Function  TreatAsAtomicUnit=on
  Scale_Roll_RC1 : MATLAB Function  TreatAsAtomicUnit=on
  Scale_Throttle_RC : MATLAB Function  TreatAsAtomicUnit=on
  Scale_Throttle_RC1 : MATLAB Function  TreatAsAtomicUnit=on
  Scale_Yaw_RC : MATLAB Function  TreatAsAtomicUnit=on
  TARGET_OUT : Outport
  wires:
  RC_IN/1 -> Bus Selector1/1, Bus Selector5/1
  Bus Selector5/4 -> Scale_Yaw_RC/1(RC_Yaw)  "<Rc_Yaw>"
  Bus Selector5/3 -> Scale_Pitch_RC/1(RC_Pitch)  "<Rc_Pitch>"
  Bus Selector5/2 -> Scale_Roll_RC/1(RC_Roll)  "<Rc_Roll>"
  Bus Selector5/1 -> Scale_Throttle_RC/1(RC_Throttle)  "<Rc_Thrust>"
  Scale_Roll_RC/1(T_ROLL) -> Mux/1  "T_ROLL"
  Bus Creator/1 -> TARGET_OUT/1
  Scale_Throttle_RC/1(T_THROTTLE) -> PWM2THRUST/1(THROTTLE_CONTROL_INPUT)
  Scale_Pitch_RC/1(T_PITCH) -> Mux/2  "T_PITCH"
  Scale_Yaw_RC/1(T_YAW) -> Mux/3  "T_YAW"
  Discrete Derivative/1 -> Bus Creator/8  "T_RATE_THROTTLE"
  Discrete Derivative1/1 -> Bus Creator/9  "T_RATE_ROLL"
  Discrete Derivative2/1 -> Bus Creator/10  "T_RATE_PITCH"
  Discrete Derivative3/1 -> Bus Creator/11  "T_RATE_YAW"
  PWM2THRUST/1(THROTTLE_CONTROL_OUTPUT) -> Discrete LowPassFilter Roll/1  "T_THROTTLE"
  Discrete LowPassFilter Roll/1 -> Discrete Derivative/1, Bus Creator/1  "T_THROTTLE"
  Discrete LowPassFilter Roll1/1 -> Discrete Derivative1/1, Bus Creator/2  "T_ROLL"
  Discrete LowPassFilter Roll2/1 -> Discrete Derivative2/1, Bus Creator/3  "T_PITCH"
  Discrete LowPassFilter Roll3/1 -> Discrete Derivative3/1, Bus Creator/4  "T_YAW"
  RC_REF_BIAS/1(RC_OUT) -> Demux/1
  Demux/1 -> Discrete LowPassFilter Roll1/1
  Demux/2 -> Discrete LowPassFilter Roll2/1
  Demux/3 -> Discrete LowPassFilter Roll3/1
  Mux/1 -> RC_REF_BIAS/1(RC_IN)
  SYSTEM_MODE_IN/1 -> Bus Selector2/1
  Bus Selector2/1 -> Logical Operator2/1  "<ARM_CMD>"
  Logical Operator3/1 -> RC_REF_BIAS/2(CONFIG_CMD)
  Logical Operator2/1 -> Logical Operator5/1, Logical Operator3/1
  Bus Selector2/2 -> Logical Operator4/1, Logical Operator3/2  "<PRE_ARM_CMD>"
  Logical Operator5/1 -> Discrete LowPassFilter Roll6/2, Discrete LowPassFilter Roll5/2, Discrete LowPassFilter Roll4/2, Discrete LowPassFilter Roll/2, Discrete LowPassFilter Roll1/2, Discrete LowPassFilter Roll2/2, Discrete LowPassFilter Roll3/2, RC_REF_BIAS/3(RESET)
  Logical Operator4/1 -> Logical Operator5/2
  Discrete LowPassFilter Roll4/1 -> Discrete Derivative4/1, Bus Creator/5  "T_X"
  Discrete LowPassFilter Roll5/1 -> Discrete Derivative5/1, Bus Creator/6  "T_Y"
  Discrete LowPassFilter Roll6/1 -> Discrete Derivative6/1, Bus Creator/7  "T_Z"
  Discrete Derivative4/1 -> Bus Creator/12  "T_RATE_X"
  Discrete Derivative5/1 -> Bus Creator/13  "T_RATE_Y"
  Discrete Derivative6/1 -> Bus Creator/14  "T_RATE_Z"
  Bus Selector1/3 -> Scale_Throttle_RC1/1(RC_Thrust)  "<Rc_Thrust>"
  Bus Selector1/1 -> Scale_Pitch_RC1/1(RC_Pitch)  "<Rc_Pitch>"
  Bus Selector1/2 -> Scale_Roll_RC1/1(RC_Roll)  "<Rc_Roll>"
  Scale_Pitch_RC1/1(T_X) -> Mux/4
  Scale_Roll_RC1/1(T_Y) -> Mux/5
  Scale_Throttle_RC1/1(T_Z) -> Mux/6
  Demux/4 -> Discrete LowPassFilter Roll4/1
  Demux/5 -> Discrete LowPassFilter Roll5/1
  Demux/6 -> Discrete LowPassFilter Roll6/1

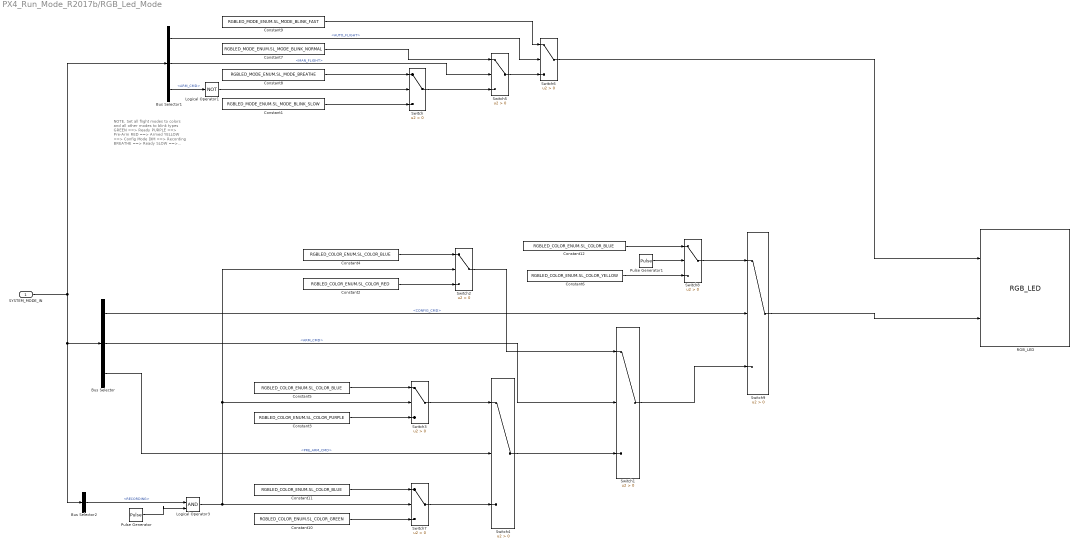
== system PX4_Run_Mode_R2017b/RGB_Led_Mode ==
  note: NOTE, Set all flight modes to colors
      | and all other modes to blink types
      |
      | GREEN		==>		Ready
      | PURPLE  	==>		Pre-Arm
      | RED		==>		Armed
      | YELLOW	==>		Config Mode
      |
      | DIM			==>		Recording
      |
      | BREATHE	==>		Ready
      | SLOW		==>		Armed MAN
      | NORMAL	==>		Armed AUTO
  SYSTEM_MODE_IN : Inport
  Bus Selector : BusSelector  OutputSignals=CONFIG_CMD,ARM_CMD,PRE_ARM_CMD
  Bus Selector1 : BusSelector  OutputSignals=AUTO_FLIGHT,MAN_FLIGHT,ARM_CMD
  Bus Selector2 : BusSelector  OutputSignals=RECORDING
  Constant1 : Constant  Value=RGBLED_MODE_ENUM.SL_MODE_BLINK_SLOW  SampleTime=Ts
  Constant10 : Constant  Value=RGBLED_COLOR_ENUM.SL_COLOR_GREEN  SampleTime=Ts
  Constant{4..5,11..12} (4 alike) : Constant  Value=RGBLED_COLOR_ENUM.SL_COLOR_BLUE  SampleTime=Ts
  Constant2 : Constant  Value=RGBLED_COLOR_ENUM.SL_COLOR_RED  SampleTime=Ts
  Constant3 : Constant  Value=RGBLED_COLOR_ENUM.SL_COLOR_PURPLE  SampleTime=Ts
  Constant6 : Constant  Value=RGBLED_COLOR_ENUM.SL_COLOR_YELLOW  SampleTime=Ts
  Constant7 : Constant  Value=RGBLED_MODE_ENUM.SL_MODE_BLINK_NORMAL  SampleTime=Ts
  Constant8 : Constant  Value=RGBLED_MODE_ENUM.SL_MODE_BREATHE  SampleTime=Ts
  Constant9 : Constant  Value=RGBLED_MODE_ENUM.SL_MODE_BLINK_FAST  SampleTime=Ts
  Logical Operator1 : Logic  Operator=NOT  IconShape=distinctive  AllPortsSameDT=off  OutDataTypeStr=boolean
  Logical Operator3 : Logic  IconShape=distinctive  AllPortsSameDT=off  OutDataTypeStr=boolean
  Pulse Generator : DiscretePulseGenerator  Period=400  PulseWidth=200  SampleTime=Ts
  Pulse Generator1 : DiscretePulseGenerator  Period=400  PulseWidth=200  SampleTime=Ts
  RGB_LED : pixhawk_slib_sensors_actuators/RGB_LED
      settings: SourceProductName=Pixhawk Target Blocks
  Switch{,1..9} (10 alike) : Switch  Criteria=u2 > Threshold
  wires:
  Bus Selector/3 -> Switch4/2  "<PRE_ARM_CMD>"
  Switch/1 -> Switch5/3
  Bus Selector1/2 -> Switch5/2  "<MAN_FLIGHT>"
  Constant7/1 -> Switch5/1
  Switch5/1 -> Switch6/3
  Bus Selector1/1 -> Switch6/2  "<AUTO_FLIGHT>"
  Constant9/1 -> Switch6/1
  Switch6/1 -> RGB_LED/1
  Switch7/1 -> Switch4/3
  Switch3/1 -> Switch4/1
  Switch4/1 -> Switch1/3
  Bus Selector/2 -> Switch1/2  "<ARM_CMD>"
  Switch2/1 -> Switch1/1
  Switch9/1 -> RGB_LED/2
  Switch1/1 -> Switch9/3
  Switch8/1 -> Switch9/1
  Bus Selector/1 -> Switch9/2  "<CONFIG_CMD>"
  Constant11/1 -> Switch7/1
  Constant10/1 -> Switch7/3
  Constant5/1 -> Switch3/1
  Constant3/1 -> Switch3/3
  Constant2/1 -> Switch2/3
  Constant4/1 -> Switch2/1
  Constant12/1 -> Switch8/1
  Constant6/1 -> Switch8/3
  Bus Selector1/3 -> Logical Operator1/1  "<ARM_CMD>"
  Logical Operator1/1 -> Switch/2
  Constant8/1 -> Switch/1
  Constant1/1 -> Switch/3
  Logical Operator3/1 -> Switch3/2, Switch2/2, Switch7/2
  Bus Selector2/1 -> Logical Operator3/1  "<RECORDING>"
  Pulse Generator/1 -> Logical Operator3/2
  Pulse Generator1/1 -> Switch8/2
  SYSTEM_MODE_IN/1 -> Bus Selector2/1, Bus Selector/1, Bus Selector1/1

== system PX4_Run_Mode_R2017b/SENSORS ==
  Battery : Subsystem
  Create Busses : Subsystem
  GPS : Subsystem
  Sensor_Combined : Subsystem
  Sonar : Subsystem
  RAW_SENSOR_DATA_OUT : Outport
  tag scope: CLOCKS=global, RAW_SENSOR_DATA=global
  wires:
  Sonar/1(RAW_SENSOR_DATA_OUT) -> [RAW_SENSOR_DATA], RAW_SENSOR_DATA_OUT/1
  Create Busses/2(TIME_OUT) -> Sensor_Combined/2(TIME_IN)
  Create Busses/1(RAW_SENSOR_DATA_OUT) -> Sensor_Combined/1(RAW_SENSOR_DATA_IN)
  Sensor_Combined/2(TIME_OUT) -> GPS/2(TIME_IN)
  Sensor_Combined/1(RAW_SENSOR_DATA_OUT) -> GPS/1(RAW_SENSOR_DATA_IN)
  GPS/1(RAW_SENSOR_DATA_OUT) -> Battery/1(RAW_SENSOR_DATA_IN)
  GPS/2(TIME_OUT) -> Battery/2(TIME_IN)
  Battery/1(RAW_SENSOR_DATA_OUT) -> Sonar/1(RAW_SENSOR_DATA_IN)
  Battery/2(TIME_OUT) -> Sonar/2(TIME_IN)
  Sonar/2(TIME_OUT) -> [CLOCKS]

== system PX4_Run_Mode_R2017b/SENSOR_FILTER ==
  RAW_SENSOR_DATA_IN : Inport
  SYSTEM_MODE_IN : Inport  Port=2
  Bias Removal State : Subsystem
  Bus Assignment : BusAssignment  AssignedSignals=Control Gains Parameters.C1,Control Gains Parameters.C2,Control Gains Parameters.C3,Control Gains Parameters.C4,Control Gains Parameters.C5,Control Gains Parameters.C6,Control Gains Parameters.C7,Control Gains Parameters.C8,Control Gains Parameters.C9,Control Gains Parameters.C10,Control Gains Parameters.C11,Control Gains Parameters.C12,Control Gains Parameters.C13,Control Gains Parameters.C14,Control Gains Parameters.C15,Control Gains Parameters.C16,Control Gains Parameters.C17,Control Gains Parameters.C18,Control Gains Parameters.C19,Control Gains Parameters.C20,Control Gains Parameters.C21,Control Gains Parameters.C22,Control Gains Parameters.C23,Control Gains Parameters.C24
  Control Gains : Constant  Value=[C1 C2 C3 C4 C5 C6 C7 C8 C9 C10 C11 C12 C13 C14 C15 C16 C17 C18 C19 C20 C21 C22 C23 C24]  OutDataTypeStr=single  SampleTime=Ts
  Demux : Demux  Outputs=24
  Fixed Bias removal and scaling : Subsystem
  SensorData2States : Subsystem
  StateEstimatesInitialConditions : Subsystem
  ESTIMATED_STATE_OUT : Outport
  tag scope: ESTIMATED_STATE=global, FILTERED_SENSOR_DATA=global, PARAMETERS=global
  wires:
  SYSTEM_MODE_IN/1 -> Fixed Bias removal and scaling/3(SYSTEM_MODE_IN), SensorData2States/3(SYSTEM_MODE), Bias Removal State/3(SYSTEM_MODE_IN)
  RAW_SENSOR_DATA_IN/1 -> Fixed Bias removal and scaling/2(RAW_SENSOR_DATA_IN)
  Bias Removal State/1(ESTIMATED_STATE_OUT) -> ESTIMATED_STATE_OUT/1, [ESTIMATED_STATE]
  StateEstimatesInitialConditions/2(FILTERED_SENSOR_DATA_OUT) -> Fixed Bias removal and scaling/1(FILTERED_SENSOR_DATA_IN)
  Fixed Bias removal and scaling/1(FILTERED_SENSOR_DATA_OUT) -> [FILTERED_SENSOR_DATA], SensorData2States/2(FILTERED_SENSOR_DATA_IN)
  StateEstimatesInitialConditions/1(ESTIMATED_STATE_OUT) -> SensorData2States/1(ESTIMATED_STATE_IN)
  Fixed Bias removal and scaling/2(PARAMETERS_OUT) -> Bias Removal State/2(PARAMETERS_IN)
  SensorData2States/1(ESTIMATED_STATE_OUT) -> Bias Removal State/1(ESTIMATED_STATE_IN)
  Bias Removal State/2(PARAMETERS_OUT) -> Bus Assignment/1
  Bus Assignment/1 -> [PARAMETERS]
  Control Gains/1 -> Demux/1
  Demux/13 -> Bus Assignment/14
  Demux/12 -> Bus Assignment/13
  Demux/14 -> Bus Assignment/15
  Demux/11 -> Bus Assignment/12
  Demux/15 -> Bus Assignment/16
  Demux/10 -> Bus Assignment/11
  Demux/16 -> Bus Assignment/17
  Demux/9 -> Bus Assignment/10
  Demux/17 -> Bus Assignment/18
  Demux/8 -> Bus Assignment/9
  Demux/18 -> Bus Assignment/19
  Demux/7 -> Bus Assignment/8
  Demux/19 -> Bus Assignment/20
  Demux/6 -> Bus Assignment/7
  Demux/20 -> Bus Assignment/21
  Demux/5 -> Bus Assignment/6
  Demux/21 -> Bus Assignment/22
  Demux/4 -> Bus Assignment/5
  Demux/22 -> Bus Assignment/23
  Demux/3 -> Bus Assignment/4
  Demux/23 -> Bus Assignment/24
  Demux/2 -> Bus Assignment/3
  Demux/24 -> Bus Assignment/25
  Demux/1 -> Bus Assignment/2

== system PX4_Run_Mode_R2017b/Speaker_Tune_Mode ==
  SYSTEM_MODE_IN : Inport
  Bus Selector : BusSelector  OutputSignals=ARM_CMD
  Constant : Constant  Value=PX4_TUNE_ENUM.ARMING_WARNING_TUNE
  Constant1 : Constant  Value=PX4_TUNE_ENUM.NOTIFY_POSITIVE_TUNE
  Data Type Conversion : DataTypeConversion  OutDataTypeStr=uint8
  Delay : Delay  DelayLength=1  InitialCondition=0
  Ground : Ground
  Logical Operator : Logic  Operator=XOR  IconShape=distinctive  AllPortsSameDT=off  OutDataTypeStr=boolean
  Speaker_Tune : pixhawk_slib_sensors_actuators/Speaker_Tune
      settings: SourceProductName=Pixhawk Target Blocks
  Switch : Switch  Criteria=u2 > Threshold
  wires:
  Ground/1 -> Speaker_Tune/2
  Switch/1 -> Speaker_Tune/1
  Constant/1 -> Switch/1
  Constant1/1 -> Switch/3
  Data Type Conversion/1 -> Speaker_Tune/3
  Logical Operator/1 -> Data Type Conversion/1
  Delay/1 -> Logical Operator/1
  SYSTEM_MODE_IN/1 -> Bus Selector/1
  Bus Selector/1 -> Delay/1, Logical Operator/2, Switch/2  "<ARM_CMD>"
